simulink library "alpha_ul"  (R2020a)
settings: Solver=VariableStepAuto  StartTime=0.0  StopTime=10.0  RelTol=1e-3
settings Model: Creator=mcobb  LastModifiedBy=John Jr
settings DataIOCC: ReturnWorkspaceOutputs=off
settings DebuggingCC: ArithmeticOperatorsInVariantConditions=warning
settings SFSimCC: CustomCodeUndefinedFunction=UseInterfaceOnly

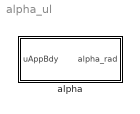
== system alpha_ul ==
  alpha : Subsystem  TreatAsAtomicUnit=on
      settings: MinAlgLoopOccurrences=on

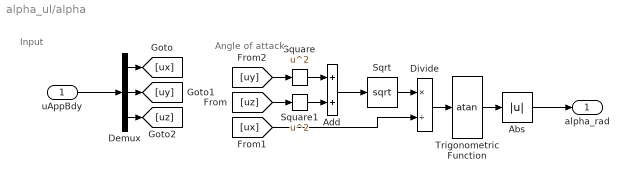
== system alpha_ul/alpha ==
  note: Angle of attack
  note: Input
  uAppBdy : Inport
  Abs : Abs
  Add : Sum
  Demux : Demux  Outputs=3
  Divide : Product  Inputs=*/
  Sqrt : Sqrt  SaturateOnIntegerOverflow=on
  Square : Math  Operator=square  SaturateOnIntegerOverflow=on
  Square1 : Math  Operator=square  SaturateOnIntegerOverflow=on
  Trigonometric Function : Trigonometry  Operator=atan
  alpha_rad : Outport  VectorParamsAs1DForOutWhenUnconnected=off
  wires:
  uAppBdy/1 -> Demux/1
  Demux/1 -> [ux]
  Demux/2 -> [uy]
  Demux/3 -> [uz]
  Trigonometric Function/1 -> Abs/1
  Divide/1 -> Trigonometric Function/1
  [ux] -> Divide/2
  [uy] -> Square/1
  [uz] -> Square1/1
  Square/1 -> Add/1
  Square1/1 -> Add/2
  Add/1 -> Sqrt/1
  Sqrt/1 -> Divide/1
  Abs/1 -> alpha_rad/1
